simulink model "cs_nonlinear"  (R2015b)
settings: Solver=ode23  StartTime=0.0  StopTime=0.1  MaxStep=4e-7  MinStep=1e-8  RelTol=1e-3
values from neighbouring files (symbols this model uses):
  c = 6e5    (= 600000)    [nonlinear.m]
  Iref = 10    [nonlinear.m]
  Ki = 0    [nonlinear.m]
undefined symbols (not defined in the file or in its folder): f_sw
libraries: powerlib x16
settings Model: Creator=Akshay  LastModifiedBy=Akshay
settings SolverCC: ZeroCrossAlgorithm=Adaptive
settings DataIOCC: LimitDataPoints=off  SaveFormat=StructureWithTime
settings HardwareCC: ProdWordSize=32  ProdHWDeviceType=Specified

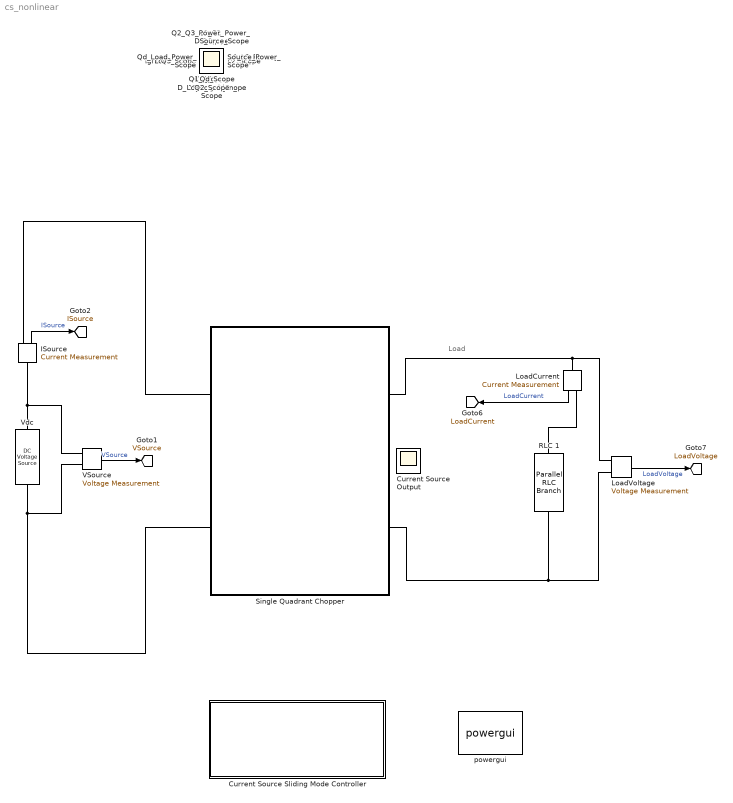
== system cs_nonlinear ==
  note: Load
  " RLC 1" : powerlib/Elements/Parallel RLC Branch  LConnTagsString=a  RConnTagsString=__new0  BranchType=R  Resistance=1  Inductance=1e-3  SetiL0=off  InitialCurrent=0  Capacitance=0.1e-6  Setx0=off  InitialVoltage=0  Measurements=None
  Current Source Output : Scope
      settings: Floating=on
  Current Source Sliding Mode Controller : Subsystem
  ISource : powerlib/Measurements/Current Measurement  PhasorSimulation=off  OutputType=Complex  PSBequivalent=0
  LoadCurrent : powerlib/Measurements/Current Measurement  PhasorSimulation=off  OutputType=Complex  PSBequivalent=0
  LoadVoltage : powerlib/Measurements/Voltage Measurement  PhasorSimulation=off  OutputType=Complex  PSBequivalent=0
  Single Quadrant Chopper : Subsystem
  VSource : powerlib/Measurements/Voltage Measurement  PhasorSimulation=off  OutputType=Complex  PSBequivalent=0
  Vdc : powerlib/Electrical Sources/DC Voltage Source  Amplitude=100  Measurements=Voltage
  powergui : powerlib/powergui  Priority=1  SimulationMode=Continuous  SolverType=Backward Euler  SampleTime=0.01/f_sw  frequency=60  SPID=on  DisableSnubberDevices=off  DisableRonSwitches=off  DisableVfSwitches=off  SwTol=0  DisplayEquations=off  Interpol=off  ExternalGateDelay=off  methode=off  Ts=0  FunctionMessages=off  echomessages=off  HookPort=off  EnableUseOfTLC=off  x0status=zero  frequencyindice=0  Pbase=100e6  ErrMax=1e-4  Iterations=50  UnitsV=kV  UnitsW=MW  buscounter=0  RestoreLinks=warning  ResistiveCurrentMeasurement=off  Frange=[0:2:500]  Ylog=off  Xlog=on  ShowGrid=off  save=off  variable=ZData  structure=ScopeData  ZoomFFT=off  StartTime=0.0  cycles=5  DisplayStyle=2  fundamental=50  FreqAxis=off  MaxFrequency=50000  frequencyindicesteady=1  RmsSteady=1  display=off
  C2_Scope : Scope
  D1_Scope : Scope
  D_D1_Power_Scope : Scope
  D_Scope : Scope
  Ignition_Scope : Scope
  L1_C2_Power_Scope : Scope
  L1_Scope : Scope
  L2_Scope : Scope
  Load_Ignition_Scope : Scope
  Load_Scope : Scope
  Q1_L2_Power_Scope : Scope
  Q1_Scope : Scope
  Q2_Q3_Power_Scope : Scope
  Q2_Scope : Scope
  Q3_Scope : Scope
  Qd_Load_Power_Scope : Scope
  Qd_Scope : Scope
  Source_Power_Scope : Scope
  Source_Scope : Scope
  tag scope: ISource=global, LoadCurrent=global, LoadVoltage=global, VSource=global
  wires:
  LoadCurrent/1 -> [LoadCurrent]  "LoadCurrent"
  LoadVoltage/1 -> [LoadVoltage]  "LoadVoltage"
  VSource/1 -> [VSource]  "VSource"
  ISource/1 -> [ISource]  "ISource"
  connections:
  LoadCurrent/RConn1 -- " RLC 1"/LConn1
  LoadVoltage/LConn1 -- Single Quadrant Chopper/RConn1 -- LoadCurrent/LConn1
  ISource/RConn1 -- Single Quadrant Chopper/LConn1
  Single Quadrant Chopper/LConn2 -- VSource/LConn2 -- Vdc/LConn1
  LoadVoltage/LConn2 -- Single Quadrant Chopper/RConn2 -- " RLC 1"/RConn1
  ISource/LConn1 -- Vdc/RConn1 -- VSource/LConn1

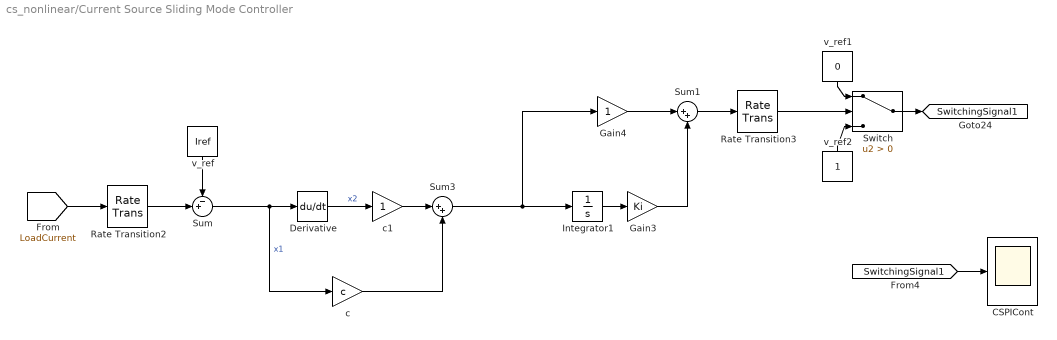
== system cs_nonlinear/Current Source Sliding Mode Controller ==
  CSPICont : Scope
  Derivative : Derivative
  Gain3 : Gain  Gain=Ki
  Gain4 : Gain
  Integrator1 : Integrator  ZeroCross=off
  Rate Transition2 : RateTransition  OutPortSampleTime=0.5/50e3
  Rate Transition3 : RateTransition  OutPortSampleTime=0.5/50e3
  Sum : Sum  Inputs=-+|
  Sum1 : Sum  Inputs=|++
  Sum3 : Sum  Inputs=|++
  Switch : Switch  Criteria=u2 > Threshold  ZeroCross=off
  c : Gain  Gain=c
  c1 : Gain
  v_ref : Constant  Value=Iref
  v_ref1 : Constant  Value=0
  v_ref2 : Constant
  tag scope: SwitchingSignal1=global
  wires:
  v_ref/1 -> Sum/1
  v_ref2/1 -> Switch/3
  v_ref1/1 -> Switch/1
  Switch/1 -> [SwitchingSignal1]
  [SwitchingSignal1] -> CSPICont/1
  Sum/1 -> c/1, Derivative/1  "x1"
  c/1 -> Sum3/2
  [LoadCurrent] -> Rate Transition2/1
  Rate Transition2/1 -> Sum/2
  Integrator1/1 -> Gain3/1
  Sum3/1 -> Gain4/1, Integrator1/1
  Gain4/1 -> Sum1/1
  Gain3/1 -> Sum1/2
  Sum1/1 -> Rate Transition3/1
  Rate Transition3/1 -> Switch/2
  c1/1 -> Sum3/1
  Derivative/1 -> c1/1  "x2"

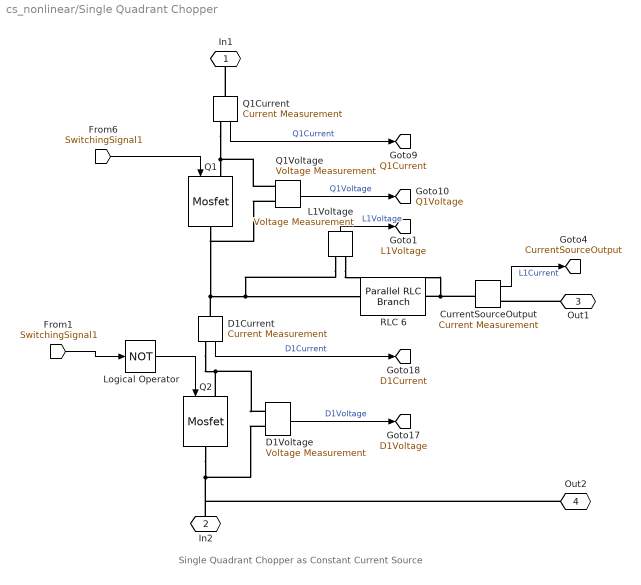
== system cs_nonlinear/Single Quadrant Chopper ==
  note: Single Quadrant Chopper as Constant Current Source
  " RLC 6" : powerlib/Elements/Parallel RLC Branch  LConnTagsString=a  RConnTagsString=__new0  BranchType=L  Resistance=50  Inductance=2e-3  SetiL0=off  InitialCurrent=100  Capacitance=0.3e-6  Setx0=off  InitialVoltage=0  Measurements=None
  CurrentSourceOutput : powerlib/Measurements/Current Measurement  PhasorSimulation=off  OutputType=Complex  PSBequivalent=0
  D1Current : powerlib/Measurements/Current Measurement  PhasorSimulation=off  OutputType=Complex  PSBequivalent=0
  D1Voltage : powerlib/Measurements/Voltage Measurement  PhasorSimulation=off  OutputType=Complex  PSBequivalent=0
  "L1Voltage " : powerlib/Measurements/Voltage Measurement  PhasorSimulation=off  OutputType=Complex  PSBequivalent=0
  Logical Operator : Logic  Operator=NOT  AllPortsSameDT=off  OutDataTypeStr=boolean
  Q1 : powerlib/Power Electronics/Mosfet  Ron=0.1  Lon=0  Rd=0.01  Vfd=0  IC=0  Rs=1e5  Cs=inf  Measurements=off
  Q1Current : powerlib/Measurements/Current Measurement  PhasorSimulation=off  OutputType=Complex  PSBequivalent=0
  Q1Voltage : powerlib/Measurements/Voltage Measurement  PhasorSimulation=off  OutputType=Complex  PSBequivalent=0
  Q2 : powerlib/Power Electronics/Mosfet  Ron=0.1  Lon=0  Rd=0.01  Vfd=0  IC=0  Rs=1e5  Cs=inf  Measurements=off
  In1 : PMIOPort  Port=1  Side=Left
  In2 : PMIOPort  Port=2  Side=Left
  Out1 : PMIOPort  Port=3  Side=Right
  Out2 : PMIOPort  Port=4  Side=Right
  tag scope: CurrentSourceOutput=global, D1Current=global, D1Voltage=global, L1Voltage=global, Q1Current=global, Q1Voltage=global
  wires:
  CurrentSourceOutput/1 -> [CurrentSourceOutput]  "L1Current"
  [SwitchingSignal1] -> Q1/1
  Q1Current/1 -> [Q1Current]  "Q1Current"
  Q1Voltage/1 -> [Q1Voltage]  "Q1Voltage"
  D1Current/1 -> [D1Current]  "D1Current"
  D1Voltage/1 -> [D1Voltage]  "D1Voltage"
  "L1Voltage "/1 -> [L1Voltage]  "L1Voltage"
  Logical Operator/1 -> Q2/1
  [SwitchingSignal1] -> Logical Operator/1
  connections:
  Q1Current/LConn1 -- In1/RConn1
  Q1Voltage/LConn2 -- Q1/RConn1 -- D1Current/LConn1 -- " RLC 6"/LConn1 -- "L1Voltage "/LConn1
  CurrentSourceOutput/LConn1 -- "L1Voltage "/LConn2 -- " RLC 6"/RConn1
  Q1Current/RConn1 -- Q1Voltage/LConn1 -- Q1/LConn1
  D1Current/RConn1 -- Q2/LConn1 -- D1Voltage/LConn1
  D1Voltage/LConn2 -- Q2/RConn1 -- Out2/RConn1 -- In2/RConn1
  Out1/RConn1 -- CurrentSourceOutput/RConn1
